simulink model "prob1"  (R2020b)
settings: Solver=VariableStepAuto  StartTime=0.0  StopTime=10.0  RelTol=1e-3
settings Model: Creator=DELL  LastModifiedBy=DELL

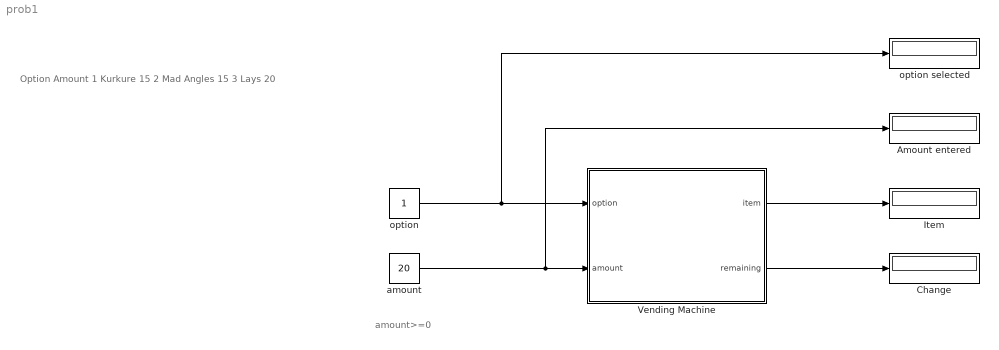
== system prob1 ==
  note: amount>=0
  note: Option
      |
      | Amount
      |
      | 1
      | Kurkure
      | 15
      |
      | 2
      | Mad Angles
      | 15
      |
      | 3
      | Lays
      | 20
  Amount entered : Display
  Change : Display
  Item : Display
  Vending Machine : Stateflow chart  TreatAsAtomicUnit=on
  amount : Constant  Value=20
  option : Constant
  option selected : Display
  wires:
  option/1 -> option selected/1, Vending Machine/1(option)
  amount/1 -> Amount entered/1, Vending Machine/2(amount)
  Vending Machine/2(remaining) -> Change/1
  Vending Machine/1(item) -> Item/1

== stateflow chart prob1/Vending Machine ==
  state Start
  state Kurkure
  state Lays
  state Mad_Angles
  state Bank3
  state Bank1
  state Bank2
  state Release
  Release -> Start : [amount<15]
      | {item=0;money=0;remaining=0;}
  (default) -> Start
  Start -> Kurkure [order 1] : [option==1]
  Start -> Lays [order 3] : [option==3]
  Start -> Mad_Angles [order 2] : [option==2]
  Kurkure -> Bank1 : {money=money+amount;}
  Bank1 -> Kurkure [order 1] : [money<15]
  Bank3 -> Lays [order 1] : [money<20]
  Lays -> Bank3 : {money=money+amount;}
  Bank2 -> Mad_Angles [order 1] : [money<15]
  Mad_Angles -> Bank2 : {money=money+amount;}
  Bank3 -> Release [order 2] : [money>=20]
      | {item=3;
      | remaining=money-20;}
  Bank2 -> Release [order 2] : [money>=15]
      | {item=2;
      | remaining=money-15;}
  Bank1 -> Release [order 2] : [money>=15]
      | {item=1;
      | remaining=money-15;}
  data: option input; amount input; item output; remaining output; money local =0
